simulink model "3-Phase Diode Rectifier"  (R2025a)
settings: Solver=VariableStepAuto  StartTime=0.0  StopTime=100  RelTol=1e-3
values from neighbouring files (symbols this model uses):
  OnTime = (SpikeTime / TimePeriod) * 100    [run_week_6_day_4.m]
  SpikeTime = evalin('base', 'SpikeTime')    [run_week_6_day_4.m]
  TimePeriod = evalin('base', 'TimePeriod')    [run_week_6_day_4.m]
undefined symbols (not defined in the file or in its folder): myFlag
libraries: fl_lib x32, nesl_utility x22, ee_lib x11
settings Model: Creator=adars  LastModifiedBy=adars
settings DebuggingCC: AlgebraicLoopMsg=none

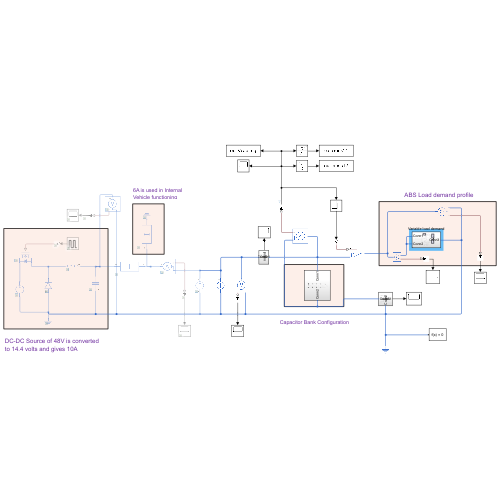
[thumbnail: Simulink's stored preview of the top-level diagram]
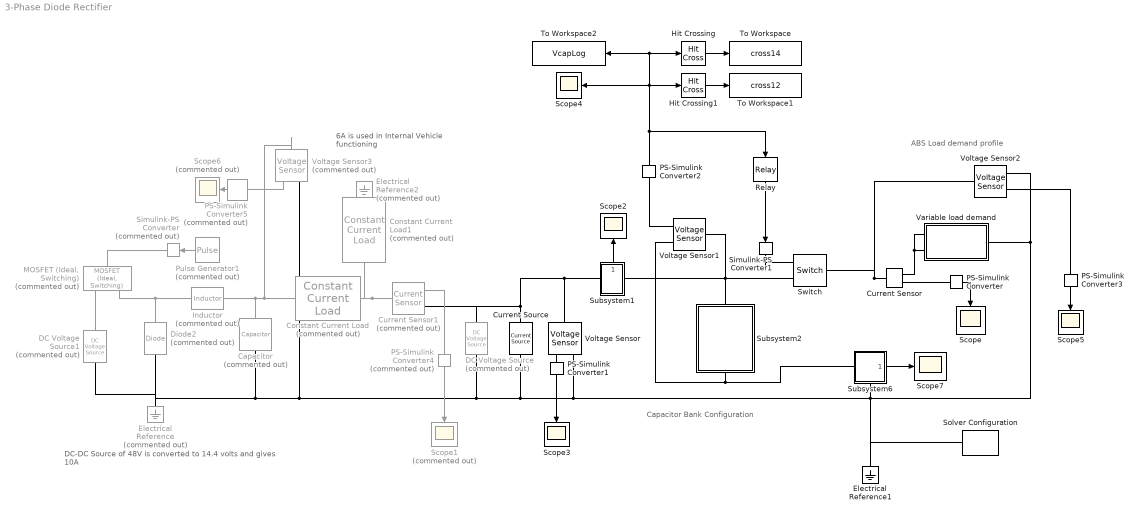
== system 3-Phase Diode Rectifier ==
  note: Capacitor Bank Configuration
  note: ABS Load demand profile
  note: 6A is used in Internal
      | Vehicle functioning
  note: DC-DC Source of 48V is converted
      | to 14.4 volts and gives 10A
  Capacitor : fl_lib/Electrical/Electrical Elements/Capacitor  Commented=on  c=48.3e-6 F  r=1e-6 Ohm  g=0 1/Ohm  i_specify=off  i_priority=None  i=0 A  i_nominal_specify=off  i_nominal_value=1  i_nominal_unit=A  v_specify=off  v_priority=None  v=0 V  v_nominal_specify=off  v_nominal_value=1  v_nominal_unit=V  vc_specify=off  vc_priority=High  vc=0 V  vc_nominal_specify=off  vc_nominal_value=1  vc_nominal_unit=V
  Constant Current Load : ee_lib/Passive/Constant Current Load  Commented=on  load_type=ee.enum.dc_ac.dc  consumed_current=10 A  min_supply_voltage=0.1 V  G_reverse=1e-6 S  deltaV=1e-3 V  consumed_current_rms=100 A  f0=60 Hz  Vrms_min=200 V
      settings: InternalSimscapePortConfiguration="{\"Bottom\":[],\"Left\":[{\"id\":\"p\",\"label\":\"+\",\"type\":\"foundation.electrical.electrical\"}],\"Right\":[{\"id\":\"n\",\"label\":\"-\",\"type\":\"foundation.electrical.electrical\"}],\"Top\":[]}"
  Constant Current Load1 : ee_lib/Passive/Constant Current Load  Commented=on  load_type=ee.enum.dc_ac.dc  consumed_current=6 A  min_supply_voltage=5 V  G_reverse=1e-6 S  deltaV=1e-3 V  consumed_current_rms=100 A  f0=60 Hz  Vrms_min=200 V
      settings: InternalSimscapePortConfiguration="{\"Bottom\":[],\"Left\":[{\"id\":\"p\",\"label\":\"+\",\"type\":\"foundation.electrical.electrical\"}],\"Right\":[{\"id\":\"n\",\"label\":\"-\",\"type\":\"foundation.electrical.electrical\"}],\"Top\":[]}"
  Current Sensor : fl_lib/Electrical/Electrical Sensors/Current Sensor
  Current Sensor1 : fl_lib/Electrical/Electrical Sensors/Current Sensor  Commented=on
  Current Source : ee_lib/Sources/Current Source  dc_current=CurrentSource A  ac_current=0 A  ac_shift=0 rad  ac_frequency=0 Hz  noise_mode=ee.enum.sources.noise.Disabled  PSD=0 A^2/Hz  sample_time=1e-3 s  repeatability=ee.enum.sources.repeatability.NotRepeatable  user_seed=0  auto_seed=3499211588  i_specify=off  i_priority=None  i=0 A  i_nominal_specify=off  i_nominal_value=1  i_nominal_unit=A  v_specify=off  v_priority=None  v=0 V  v_nominal_specify=off  v_nominal_value=1  v_nominal_unit=V
  DC Voltage Source : ee_lib/Additional Components/SPICE Sources/DC Voltage Source  Commented=on  DC=14.4 V
  DC Voltage Source1 : ee_lib/Additional Components/SPICE Sources/DC Voltage Source  Commented=on  DC=48 V
  Diode2 : fl_lib/Electrical/Electrical Elements/Diode  Commented=on  Vf=0.6 V  Ron=0.3 Ohm  Goff=1e-8 1/Ohm  i_specify=off  i_priority=None  i=0 A  i_nominal_specify=off  i_nominal_value=1  i_nominal_unit=A  v_specify=off  v_priority=None  v=0 V  v_nominal_specify=off  v_nominal_value=1  v_nominal_unit=V
  Electrical Reference : fl_lib/Electrical/Electrical Elements/Electrical Reference  Commented=on
  Electrical Reference1 : fl_lib/Electrical/Electrical Elements/Electrical Reference
  Electrical Reference2 : fl_lib/Electrical/Electrical Elements/Electrical Reference  Commented=on
  Hit Crossing : HitCross  HitCrossingOffset=14.4-1e-5  HitCrossingDirection=rising
  Hit Crossing1 : HitCross  HitCrossingOffset=12+1e-5  HitCrossingDirection=falling
  Inductor : ee_lib/Passive/Inductor  Commented=on  l=22e-6 H  enable_L_tol=ee.enum.toleranceApplication.none  L_tol=20  tol_distribution=ee.enum.toleranceDistribution.uniform  nSigma=4  r=0 Ohm  g=1e-9 1/Ohm  enable_operating_limits=ee.enum.enable.no  operating_limit_action=ee.enum.passive.reportOpLim.warn  max_working_current=1 A  power_rating=1 W  i_L_specify=off  i_L_priority=High  i_L=0 A  i_L_nominal_specify=off  i_L_nominal_value=1  i_L_nominal_unit=A
  "MOSFET (Ideal, Switching)" : ee_lib/Semiconductors & Converters/MOSFET (Ideal, Switching)  Commented=on  port_option=ee.enum.controlport.ps  Rds=0.01 Ohm  Goff=1e-6 1/Ohm  Vth=2 V  diode_param=ee.enum.semiconductors.protectionDiode.nodynamics  diode_Vf=0.8 V  diode_Ron=0.001 Ohm  diode_Goff=1e-5 1/Ohm  diode_C=50e-9 F  diode_iRM=-235 A  diode_iF=300 A  diode_idot=-50 A/us  diode_trr_param=ee.enum.converters.diodeReverseParam.trr_factor  diode_trr_factor=3  diode_trr=15 us  diode_Qrr=1500 s*uA  ids_specify=off  ids_priority=None  ids=0 A  ids_nominal_specify=off  ids_nominal_value=1  ids_nominal_unit=A  vds_specify=off  vds_priority=None  vds=0 V  vds_nominal_specify=off  vds_nominal_value=1  vds_nominal_unit=V  vgs_specify=off  vgs_priority=None  vgs=0 V  vgs_nominal_specify=off  vgs_nominal_value=1  vgs_nominal_unit=V  thermal_loss_option=ee.enum.converters.thermalLossOption.constantvalues  Von_data=[0, 1.8, 3.2, 6, 10, 16; 0, 2, 5.5, 9.5, 15, 25] V  Tj=[298.15, 448.15] K  Iout_data=[0, 20, 40, 60, 80, 100] A  Eon_data=[0, 55.04, 124.57, 235.53, 362.12; 0, 71.25, 161.25, 304.88, 468.75] * 1e-6 J  Eoff_data=[0, 18, 30, 56.1, 76.5; 0, 22.5, 37.5, 70.13, 95.63] * 1e-6 J  Eon_data_3D=[zeros(2, 5, 3)] J  Eoff_data_3D=[zeros(2, 5, 3)] J  Tj_loss=[298.15, 448.15] K  Iout_data_loss=[0, 10, 20, 30, 40] A  tabulateWithVds=false  Vds_loss=[0, 150, 300] V  Eon_scalar=22.86e-3 J  Eoff_scalar=17.14e-3 J  Voff=300 V  Iout_scalar=600 A  useCurrentFromPreviousCycle=false  useVoltageFromPreviousCycle=false  diodeModelType=ee.enum.converters.diodeModelType.pwl  diodeTableType=ee.enum.diode.tableType.IfMat  diode_ReverseIVType=ee.enum.diode.diodeReverseIV.constant  diode_IfMat=[.07, .12, .19, 1.75, 4.24, 7.32, 11.2; .16, .3, .72, 2.14, 4.02, 6.35, 9.12] A  diode_VfMat=[.9, 1.15, 1.25, 1.5, 1.75, 2.17, 2.6, 2.85; .58, .68, .75, 1.1, 1.38, 1.77, 2.27, 2.7] V  diode_TjVec=[25, 125] degC  diode_VfVec=[.5, .7, .9, 1.3, 1.7, 2.1, 2.5] V  diode_IfVec=[.1, .2, .5, 1, 2, 4, 7, 10] A  diode_IrMat=[1e-06, 2e-06, 5e-06, 1e-05, 2.5e-05, 5e-05, .0001; 2e-06, 5e-06, 1e-05, 4e-05, 8e-05, .0002, .0005] A  diode_VrMat=[10, 100, 200, 250, 300, 325, 350; 10, 70, 160, 220, 270, 300, 320] V  diode_VrVec=[10, 20, 40, 50, 70, 80, 100] V  diode_IrVec=[1e-06, 2e-06, 5e-06, 1e-05, 2e-05, 5e-05, .0001] A  diode_Vr=-600 V  diode_Ls=150 nH  diode_Erec=0.03 J  diode_rec_loss_model=ee.enum.diode.reverseRecoveryModel.fixed  diode_ErecVal=0 J  diode_scaleWithIandV=true  diode_ErecMat=zeros(2, 3) J  diode_TjrecVec=[298.15, 398.15] K  diode_IfrecVec=[.1, 1, 10] A  diode_IrecVal=10 A  diode_VrecVal=10 V  diode_tFilter=1 / 1000 / 100 s  separateThermalPortForDiode=false  thermal_network_parameterization=ee.enum.thermalNetworkTopology.external  Rth=[.03, .2] K/W  Rth_Cauer=[.03, .1, .2] K/W  Rth_Foster=[.08, .14, .22, .16] K/W  thermal_mass_parameterization=ee.enum.thermalNetwork.timeconstant  thermal_mass=[3, 25] J/K  thermal_mass_Cauer=[3, 10, 25] J/K  thermal_mass_Foster=[.001, .005, .05, .5] J/K  thermal_time_constant=[.1, 5] s  thermal_time_constant_Cauer=[.1, 1, 5] s  thermal_time_constant_Foster=[7e-05, .0007, .01, .08] s  thermal_mass_initial_temperatures=[25, 25] degC  thermal_mass_initial_temperatures_Cauer=[25, 25, 25] degC  junction_thermal_mass=0.1 J/K  Tvec_initial_Foster=[25, 25, 25, 25] degC  RthDiode=[.03, .2] K/W  RthCauerDiode=[.03, .1, .2] K/W  RthFosterDiode=[.03, .2] K/W  thermalMassDiode=[3, 25] J/K  thermalMassCauerDiode=[3, 10, 25] J/K  thermalMassFosterDiode=[33, 50] J/K  thermalTauDiode=[.1, 5] s  thermalTauCauerDiode=[.1, 1, 5] s  thermalTauFosterDiode=[1, 10] s  thermalMassInitTempDiode=[25, 25] degC  thermalMassInitTempCauerDiode=[25, 25, 25] degC  junctionthermalMassDiode=0.1 J/K  TVecInitialFosterDiode=[25, 25, 25, 25] degC  no_thermal_network=0  mosfet_junction_temperature_specify=off  mosfet_junction_temperature_priority=None  mosfet_junction_temperature=25 degC  mosfet_junction_temperature_nominal_specify=off  mosfet_junction_temperature_nominal_value=1  mosfet_junction_temperature_nominal_unit=degC  diode_junction_temperature_specify=off  diode_junction_temperature_priority=None  diode_junction_temperature=25 degC  diode_junction_temperature_nominal_specify=off  diode_junction_temperature_nominal_value=1  diode_junction_temperature_nominal_unit=degC  Qj_specify=off  Qj_priority=None  Qj=0 W  Qj_nominal_specify=off  Qj_nominal_value=1  Qj_nominal_unit=W  accumulatedSwitchingLosses_specify=off  accumulatedSwitchingLosses_priority=None  accumulatedSwitchingLosses=0 J
  PS-Simulink Converter{,1..3} (4 alike) : nesl_utility/PS-Simulink Converter  PhysicalDomain=network_engine_domain  SubClassName=ps_output  LeftPortType=input  RightPortType=output  PseudoPeriodic=off  Frequencies=[]  VectorFormat=inherit  Unit=inherit  AffineConversion=off
  PS-Simulink Converter4 : nesl_utility/PS-Simulink Converter  Commented=on  PhysicalDomain=network_engine_domain  SubClassName=ps_output  LeftPortType=input  RightPortType=output  PseudoPeriodic=off  Frequencies=[]  VectorFormat=inherit  Unit=inherit  AffineConversion=off
  PS-Simulink Converter5 : nesl_utility/PS-Simulink Converter  Commented=on  PhysicalDomain=network_engine_domain  SubClassName=ps_output  LeftPortType=input  RightPortType=output  PseudoPeriodic=off  Frequencies=[]  VectorFormat=inherit  Unit=inherit  AffineConversion=off
  Pulse Generator1 : DiscretePulseGenerator  Commented=on  PulseType=Time based  Amplitude=10  Period=6.8e-6  PulseWidth=35
  Relay : Relay  OnSwitchValue=14.4  OffSwitchValue=12
  Scope{,2..5,7} (6 alike) : Scope
      Scope settings: ActiveDisplayYMinimum=-1.307559668572738  ActiveDisplayYMaximum=0.60259783482282581
      Scope2 settings: ActiveDisplayYMinimum=3  ActiveDisplayYMaximum=5  DataLoggingVariableName=ScopeData2
      Scope3 settings: ActiveDisplayYMinimum=-1.84775774004581  ActiveDisplayYMaximum=16.629859660412297  DataLoggingVariableName=ScopeData3
      Scope4 settings: ActiveDisplayYMinimum=11.713414975625813  ActiveDisplayYMaximum=13.359784553943715  DataLoggingVariableName=ScopeData4
      Scope5 settings: ActiveDisplayYMinimum=-1.2935840970910446  ActiveDisplayYMaximum=16.143708233009956  DataLoggingVariableName=ScopeData5
      Scope7 settings: ActiveDisplayYMinimum=-24.12500014418708  ActiveDisplayYMaximum=7.1249998826875194  DataLoggingVariableName=ScopeData13
  Scope1 : Scope  Commented=on
      settings: ActiveDisplayYMinimum=-7.2502393778438039  ActiveDisplayYMaximum=5.2520104006562276  DataLoggingVariableName=ScopeData10
  Scope6 : Scope  Commented=on
      settings: ActiveDisplayYMinimum=-2.4456957415230445  ActiveDisplayYMaximum=22.011261673851934  DataLoggingVariableName=ScopeData14
  Simulink-PS Converter : nesl_utility/Simulink-PS Converter  Commented=on  PhysicalDomain=network_engine_domain  SubClassName=ps_input  LeftPortType=input  RightPortType=output  PseudoPeriodic=off  Frequencies=[]  NoiseDistribution=none  NoiseParameters=[]  Unit=1  AffineConversion=off  FilteringAndDerivatives=provide  SimscapeFilterOrder=1  InputFilterTimeConstant=0.001  UdotUserProvided=0
  Simulink-PS Converter1 : nesl_utility/Simulink-PS Converter  PhysicalDomain=network_engine_domain  SubClassName=ps_input  LeftPortType=input  RightPortType=output  PseudoPeriodic=off  Frequencies=[]  NoiseDistribution=none  NoiseParameters=[]  Unit=1  AffineConversion=off  FilteringAndDerivatives=provide  SimscapeFilterOrder=1  InputFilterTimeConstant=0.001  UdotUserProvided=0
  Solver Configuration : nesl_utility/Solver Configuration  PhysicalDomain=network_engine_domain  SubClassName=solver  LeftPortType=input  RightPortType=generic  Tones=[]  Harmonics=[]  SimulateNoise=off  Profile=off  UseLocalSampling=off  EnableSwitchedLinearOptims=on  FrequencyDomain=off  UseCCode=off  RelTol=0.001  AbsTol=0.001  MinStep=1e-09  ToWorkspace=off  RevertToSquareIcSolve=off  NumHomotopyIterations=100  PhasorMode=off  PhasorModeNumHarmonics=1  ConsistencySolver=NEWTON_XTOL_AFTER_FTOL  IndexReductionMethod=DerivativeReplacement  DoDC=off  ResidualTolerance=1e-09  ConsistencyTolSource=GLOBAL  ConsistencyAbsTol=0.001  ConsistencyRelTol=0.001  ConsistencyTolFactor=0.001  UseLocalSolver=off  LocalSolverChoice=NE_BACKWARD_EULER_ADVANCER  ResolveIndetEquations=on  FunctionEvalNumThread=1  LocalSolverSampleTime=0.001  DoFixedCost=off  MaxNonlinIter=3  MaxModeIter=2  ComputeImpulses=off  ImpulseIterations=2  LinearAlgebra=auto  LinearAlgebraNumThread=0  EquationFormulation=NE_TIME_EF  DelaysMemoryBudget=1024  AutomaticFiltering=on  FilteringTimeConstant=0.001  PartitionStorageMethod=AS_NEEDED  PartitionMemoryBudget=1024  PartitionMethod=ROBUST  MultibodyUseLocalSolver=off  MultibodyLocalSolverChoice=ODE1  MultibodyLocalSolverSampleTime=0.001
  Subsystem1 : Subsystem
      settings: PortSchema="{\"entries\":[{\"content\":{\"sides\":[{\"content\":{\"connectorIds\":[\"LConn1\"]},\"type\":\"ConnectorPlacement.EquallySpacedRectSide\",\"uuid\":\"0bfba3d8-eada-431e-8566-6f8409c961ce\"},{\"content\":{\"connectorIds\":[\"RConn1\"],\"side\":\"RIGHT\"},\"type\":\"ConnectorPlacement.EquallySpacedRectSide\",\"uuid\":\"a4875283-c2aa-4032-81af-fd742f95824b\"},{\"content\":{\"connectorIds\":[\"Out1\"],\"side\":\"TOP\"},\"type\":\"ConnectorPlacement.EquallySpacedRectSide\",\"uuid\":\"06f00768-eb41-4938-823b-845aa4a9ac6f\"}]},\"type\":\"ConnectorPlacement.EquallySpacedConnector\",\"uuid\":\"d87aa723-8170-4005-95e2-aec9f879c413\"}],\"packageUris\":[\"http://schema.mathworks.com/mf0/Connector/R2020b\"],\"version\":\"1.0\"}"
  Subsystem2 : Subsystem
  Subsystem6 : Subsystem
      settings: PortSchema="{\"entries\":[{\"content\":{\"sides\":[{\"content\":{\"connectorIds\":[\"LConn1\"]},\"type\":\"ConnectorPlacement.EquallySpacedRectSide\",\"uuid\":\"0bfba3d8-eada-431e-8566-6f8409c961ce\"},{\"content\":{\"connectorIds\":[\"Out1\"],\"side\":\"RIGHT\"},\"type\":\"ConnectorPlacement.EquallySpacedRectSide\",\"uuid\":\"a4875283-c2aa-4032-81af-fd742f95824b\"},{\"content\":{\"side\":\"TOP\"},\"type\":\"ConnectorPlacement.EquallySpacedRectSide\",\"uuid\":\"06f00768-eb41-4938-823b-845aa4a9ac6f\"},{\"content\":{\"connectorIds\":[\"RConn1\"],\"side\":\"BOTTOM\"},\"type\":\"ConnectorPlacement.EquallySpacedRectSide\",\"uuid\":\"36f95f34-d0b9-4c5e-948a-2f9aa4eedbf8\"}]},\"type\":\"ConnectorPlacement.EquallySpacedConnector\",\"uuid\":\"d87aa723-8170-4005-95e2-aec9f879c413\"}],\"packageUris\":[\"http://schema.mathworks.com/mf0/Connector/R2020b\"],\"version\":\"1.0\"}"
  Switch : fl_lib/Electrical/Electrical Elements/Switch  R_closed=0.01 Ohm  G_open=1e-8 1/Ohm  Threshold=0.5  i_specify=off  i_priority=None  i=0 A  i_nominal_specify=off  i_nominal_value=1  i_nominal_unit=A  v_specify=off  v_priority=None  v=0 V  v_nominal_specify=off  v_nominal_value=1  v_nominal_unit=V
  To Workspace : ToWorkspace  VariableName=cross14  SampleTime=-1
  To Workspace1 : ToWorkspace  VariableName=cross12  SampleTime=-1
  To Workspace2 : ToWorkspace  VariableName=VcapLog  SaveFormat=Timeseries  SampleTime=-1
  Variable load demand : Subsystem
  Voltage Sensor : fl_lib/Electrical/Electrical Sensors/Voltage Sensor
  Voltage Sensor1 : fl_lib/Electrical/Electrical Sensors/Voltage Sensor
  Voltage Sensor2 : fl_lib/Electrical/Electrical Sensors/Voltage Sensor
  Voltage Sensor3 : fl_lib/Electrical/Electrical Sensors/Voltage Sensor  Commented=on
  wires:
  PS-Simulink Converter3/1 -> Scope5/1
  PS-Simulink Converter/1 -> Scope/1
  PS-Simulink Converter5/1 -> Scope6/1
  PS-Simulink Converter1/1 -> Scope3/1
  Pulse Generator1/1 -> Simulink-PS Converter/1
  PS-Simulink Converter2/1 -> Scope4/1, To Workspace2/1, Hit Crossing/1, Hit Crossing1/1, Relay/1
  Hit Crossing1/1 -> To Workspace1/1
  Subsystem1/1(output) -> Scope2/1
  Subsystem6/1(output) -> Scope7/1
  PS-Simulink Converter4/1 -> Scope1/1
  Relay/1 -> Simulink-PS Converter1/1
  Hit Crossing/1 -> To Workspace/1
  connections:
  Voltage Sensor1/LConn1 -- Subsystem1/RConn1 -- Subsystem2/LConn1 -- Switch/RConn2
  Current Sensor/LConn1 -- Switch/LConn1 -- Voltage Sensor2/LConn1
  Diode2/RConn1 -- "MOSFET (Ideal, Switching)"/RConn2 -- Inductor/LConn1
  Constant Current Load1/LConn1 -- Constant Current Load/RConn1 -- Current Sensor1/LConn1
  Voltage Sensor3/LConn1 -- Capacitor/LConn1 -- Inductor/RConn1 -- Constant Current Load/LConn1
  Current Source/RConn1 -- Voltage Sensor3/RConn2 -- DC Voltage Source1/RConn1 -- Electrical Reference/LConn1 -- Diode2/LConn1 -- Capacitor/RConn1 -- DC Voltage Source/RConn1 -- Solver Configuration/RConn1 -- Electrical Reference1/LConn1 -- Subsystem6/RConn1 -- Voltage Sensor2/RConn2 -- Variable load demand/LConn1 -- Voltage Sensor/RConn2
  Voltage Sensor/LConn1 -- Current Sensor1/RConn2 -- DC Voltage Source/LConn1 -- Current Source/LConn1 -- Subsystem1/LConn1
  Voltage Sensor1/RConn2 -- Subsystem2/RConn1 -- Subsystem6/LConn1
  Current Sensor/RConn2 -- Variable load demand/RConn2 -- Variable load demand/RConn1
  PS-Simulink Converter1/LConn1 -- Voltage Sensor/RConn1
  PS-Simulink Converter2/LConn1 -- Voltage Sensor1/RConn1
  DC Voltage Source1/LConn1 -- "MOSFET (Ideal, Switching)"/RConn1
  PS-Simulink Converter/LConn1 -- Current Sensor/RConn1
  PS-Simulink Converter5/LConn1 -- Voltage Sensor3/RConn1
  Simulink-PS Converter/RConn1 -- "MOSFET (Ideal, Switching)"/LConn1
  Simulink-PS Converter1/RConn1 -- Switch/RConn1
  Constant Current Load1/RConn1 -- Electrical Reference2/LConn1
  Current Sensor1/RConn1 -- PS-Simulink Converter4/LConn1
  PS-Simulink Converter3/LConn1 -- Voltage Sensor2/RConn1

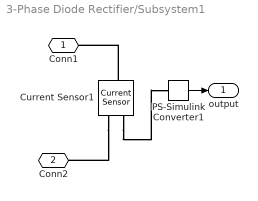
== system 3-Phase Diode Rectifier/Subsystem1 ==
  Current Sensor1 : fl_lib/Electrical/Electrical Sensors/Current Sensor
  PS-Simulink Converter1 : nesl_utility/PS-Simulink Converter  PhysicalDomain=network_engine_domain  SubClassName=ps_output  LeftPortType=input  RightPortType=output  PseudoPeriodic=off  Frequencies=[]  VectorFormat=inherit  Unit=inherit  AffineConversion=off
  Conn1 : PMIOPort  Side=Left
  Conn2 : PMIOPort  Port=2  Side=Right
  output : Outport
  wires:
  PS-Simulink Converter1/1 -> output/1
  connections:
  Current Sensor1/RConn1 -- PS-Simulink Converter1/LConn1
  Current Sensor1/LConn1 -- Conn1/RConn1
  Current Sensor1/RConn2 -- Conn2/RConn1

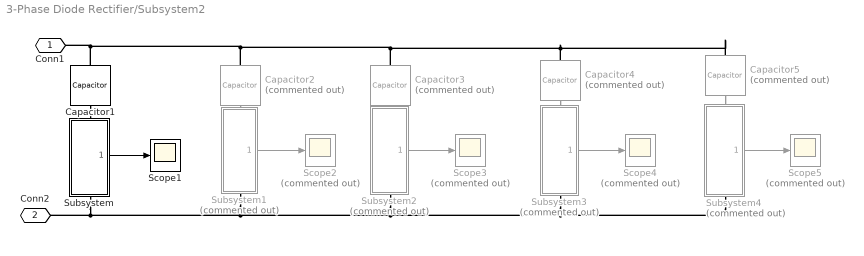
== system 3-Phase Diode Rectifier/Subsystem2 ==
  Capacitor1 : fl_lib/Electrical/Electrical Elements/Capacitor  c=C_val F  r=1e-6 Ohm  g=0 1/Ohm  i_specify=off  i_priority=None  i=0 A  i_nominal_specify=off  i_nominal_value=1  i_nominal_unit=A  v_specify=off  v_priority=None  v=0 V  v_nominal_specify=off  v_nominal_value=1  v_nominal_unit=V  vc_specify=on  vc_priority=High  vc=12 V  vc_nominal_specify=off  vc_nominal_value=1  vc_nominal_unit=V
  Capacitor{2..5} (4 alike) : fl_lib/Electrical/Electrical Elements/Capacitor  Commented=on  c=22.5 F  r=1e-6 Ohm  g=0 1/Ohm  i_specify=off  i_priority=None  i=0 A  i_nominal_specify=off  i_nominal_value=1  i_nominal_unit=A  v_specify=off  v_priority=None  v=0 V  v_nominal_specify=off  v_nominal_value=1  v_nominal_unit=V  vc_specify=on  vc_priority=High  vc=12 V  vc_nominal_specify=off  vc_nominal_value=1  vc_nominal_unit=V
  Scope1 : Scope
      settings: ActiveDisplayYMinimum=-32.03150883871016  ActiveDisplayYMaximum=5.6799472599220806
  Scope{2..5} (4 alike) : Scope  Commented=on
      Scope2 settings: ActiveDisplayYMinimum=-32.03150883871016  ActiveDisplayYMaximum=5.6799472599220806  DataLoggingVariableName=ScopeData6
      Scope3 settings: ActiveDisplayYMinimum=-32.03150883871016  ActiveDisplayYMaximum=5.6799472599220806  DataLoggingVariableName=ScopeData7
      Scope4 settings: ActiveDisplayYMinimum=-32.03150883871016  ActiveDisplayYMaximum=5.6799472599220806  DataLoggingVariableName=ScopeData8
      Scope5 settings: ActiveDisplayYMinimum=-32.03150883871016  ActiveDisplayYMaximum=5.6799472599220806  DataLoggingVariableName=ScopeData9
  Subsystem : Subsystem
      settings: PortSchema="{\"entries\":[{\"content\":{\"sides\":[{\"content\":{\"connectorIds\":[\"LConn1\"]},\"type\":\"ConnectorPlacement.EquallySpacedRectSide\",\"uuid\":\"81a8c0f4-8ed9-4d4b-bd28-04771a05fe4f\"},{\"content\":{\"connectorIds\":[\"RConn1\"],\"side\":\"RIGHT\"},\"type\":\"ConnectorPlacement.EquallySpacedRectSide\",\"uuid\":\"31ca84c7-3f86-4e13-8cf7-6dd391f2d0e6\"},{\"content\":{\"connectorIds\":[\"Out1\"],\"side\":\"TOP\"},\"type\":\"ConnectorPlacement.EquallySpacedRectSide\",\"uuid\":\"282c2d81-43af-474c-80bd-93514e90c90d\"}]},\"type\":\"ConnectorPlacement.EquallySpacedConnector\",\"uuid\":\"f82acd1c-4042-44ca-a2b0-ecaad96ae19c\"}],\"packageUris\":[\"http://schema.mathworks.com/mf0/Connector/R2020b\"],\"version\":\"1.0\"}"
  Subsystem1 : Subsystem  Commented=on
      settings: PortSchema="{\"entries\":[{\"content\":{\"sides\":[{\"content\":{\"connectorIds\":[\"LConn1\"]},\"type\":\"ConnectorPlacement.EquallySpacedRectSide\",\"uuid\":\"81a8c0f4-8ed9-4d4b-bd28-04771a05fe4f\"},{\"content\":{\"connectorIds\":[\"RConn1\"],\"side\":\"RIGHT\"},\"type\":\"ConnectorPlacement.EquallySpacedRectSide\",\"uuid\":\"31ca84c7-3f86-4e13-8cf7-6dd391f2d0e6\"},{\"content\":{\"connectorIds\":[\"Out1\"],\"side\":\"TOP\"},\"type\":\"ConnectorPlacement.EquallySpacedRectSide\",\"uuid\":\"282c2d81-43af-474c-80bd-93514e90c90d\"}]},\"type\":\"ConnectorPlacement.EquallySpacedConnector\",\"uuid\":\"f82acd1c-4042-44ca-a2b0-ecaad96ae19c\"}],\"packageUris\":[\"http://schema.mathworks.com/mf0/Connector/R2020b\"],\"version\":\"1.0\"}"
  Subsystem2 : Subsystem  Commented=on
      settings: PortSchema="{\"entries\":[{\"content\":{\"sides\":[{\"content\":{\"connectorIds\":[\"LConn1\"]},\"type\":\"ConnectorPlacement.EquallySpacedRectSide\",\"uuid\":\"81a8c0f4-8ed9-4d4b-bd28-04771a05fe4f\"},{\"content\":{\"connectorIds\":[\"RConn1\"],\"side\":\"RIGHT\"},\"type\":\"ConnectorPlacement.EquallySpacedRectSide\",\"uuid\":\"31ca84c7-3f86-4e13-8cf7-6dd391f2d0e6\"},{\"content\":{\"connectorIds\":[\"Out1\"],\"side\":\"TOP\"},\"type\":\"ConnectorPlacement.EquallySpacedRectSide\",\"uuid\":\"282c2d81-43af-474c-80bd-93514e90c90d\"}]},\"type\":\"ConnectorPlacement.EquallySpacedConnector\",\"uuid\":\"f82acd1c-4042-44ca-a2b0-ecaad96ae19c\"}],\"packageUris\":[\"http://schema.mathworks.com/mf0/Connector/R2020b\"],\"version\":\"1.0\"}"
  Subsystem3 : Subsystem  Commented=on
      settings: PortSchema="{\"entries\":[{\"content\":{\"sides\":[{\"content\":{\"connectorIds\":[\"LConn1\"]},\"type\":\"ConnectorPlacement.EquallySpacedRectSide\",\"uuid\":\"81a8c0f4-8ed9-4d4b-bd28-04771a05fe4f\"},{\"content\":{\"connectorIds\":[\"RConn1\"],\"side\":\"RIGHT\"},\"type\":\"ConnectorPlacement.EquallySpacedRectSide\",\"uuid\":\"31ca84c7-3f86-4e13-8cf7-6dd391f2d0e6\"},{\"content\":{\"connectorIds\":[\"Out1\"],\"side\":\"TOP\"},\"type\":\"ConnectorPlacement.EquallySpacedRectSide\",\"uuid\":\"282c2d81-43af-474c-80bd-93514e90c90d\"}]},\"type\":\"ConnectorPlacement.EquallySpacedConnector\",\"uuid\":\"f82acd1c-4042-44ca-a2b0-ecaad96ae19c\"}],\"packageUris\":[\"http://schema.mathworks.com/mf0/Connector/R2020b\"],\"version\":\"1.0\"}"
  Subsystem4 : Subsystem  Commented=on
      settings: PortSchema="{\"entries\":[{\"content\":{\"sides\":[{\"content\":{\"connectorIds\":[\"LConn1\"]},\"type\":\"ConnectorPlacement.EquallySpacedRectSide\",\"uuid\":\"81a8c0f4-8ed9-4d4b-bd28-04771a05fe4f\"},{\"content\":{\"connectorIds\":[\"RConn1\"],\"side\":\"RIGHT\"},\"type\":\"ConnectorPlacement.EquallySpacedRectSide\",\"uuid\":\"31ca84c7-3f86-4e13-8cf7-6dd391f2d0e6\"},{\"content\":{\"connectorIds\":[\"Out1\"],\"side\":\"TOP\"},\"type\":\"ConnectorPlacement.EquallySpacedRectSide\",\"uuid\":\"282c2d81-43af-474c-80bd-93514e90c90d\"}]},\"type\":\"ConnectorPlacement.EquallySpacedConnector\",\"uuid\":\"f82acd1c-4042-44ca-a2b0-ecaad96ae19c\"}],\"packageUris\":[\"http://schema.mathworks.com/mf0/Connector/R2020b\"],\"version\":\"1.0\"}"
  Conn1 : PMIOPort  Side=Left
  Conn2 : PMIOPort  Port=2  Side=Right
  wires:
  Subsystem/1(output) -> Scope1/1
  Subsystem1/1(output) -> Scope2/1
  Subsystem2/1(output) -> Scope3/1
  Subsystem3/1(output) -> Scope4/1
  Subsystem4/1(output) -> Scope5/1
  connections:
  Capacitor1/RConn1 -- Subsystem/LConn1
  Capacitor1/LConn1 -- Capacitor5/LConn1 -- Capacitor4/LConn1 -- Capacitor3/LConn1 -- Capacitor2/LConn1 -- Conn1/RConn1
  Subsystem/RConn1 -- Subsystem2/RConn1 -- Subsystem3/RConn1 -- Subsystem4/RConn1 -- Subsystem1/RConn1 -- Conn2/RConn1
  Capacitor2/RConn1 -- Subsystem1/LConn1
  Capacitor3/RConn1 -- Subsystem2/LConn1
  Capacitor4/RConn1 -- Subsystem3/LConn1
  Capacitor5/RConn1 -- Subsystem4/LConn1

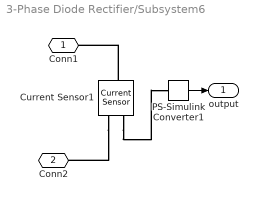
== system 3-Phase Diode Rectifier/Subsystem6 ==
  Current Sensor1 : fl_lib/Electrical/Electrical Sensors/Current Sensor
  PS-Simulink Converter1 : nesl_utility/PS-Simulink Converter  PhysicalDomain=network_engine_domain  SubClassName=ps_output  LeftPortType=input  RightPortType=output  PseudoPeriodic=off  Frequencies=[]  VectorFormat=inherit  Unit=inherit  AffineConversion=off
  Conn1 : PMIOPort  Side=Left
  Conn2 : PMIOPort  Port=2  Side=Right
  output : Outport
  wires:
  PS-Simulink Converter1/1 -> output/1
  connections:
  Current Sensor1/RConn1 -- PS-Simulink Converter1/LConn1
  Current Sensor1/LConn1 -- Conn1/RConn1
  Current Sensor1/RConn2 -- Conn2/RConn1

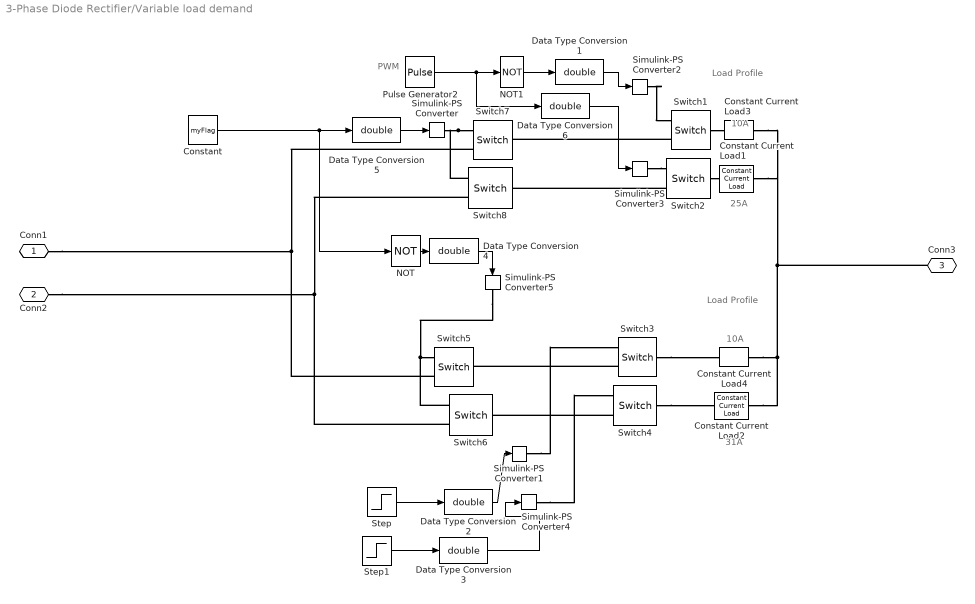
== system 3-Phase Diode Rectifier/Variable load demand ==
  note: 10A
  note: PWM
  note: 25A
  note: 10A
  note: Load Profile
  note: Load Profile
  note: 31A
  Constant : Constant  Value=myFlag
  Constant Current Load1 : ee_lib/Passive/Constant Current Load  load_type=ee.enum.dc_ac.dc  consumed_current=high_current A  min_supply_voltage=1 V  G_reverse=1e-6 S  deltaV=1e-3 V  consumed_current_rms=100 A  f0=60 Hz  Vrms_min=200 V
      settings: InternalSimscapePortConfiguration="{\"Bottom\":[],\"Left\":[{\"id\":\"p\",\"label\":\"+\",\"type\":\"foundation.electrical.electrical\"}],\"Right\":[{\"id\":\"n\",\"label\":\"-\",\"type\":\"foundation.electrical.electrical\"}],\"Top\":[]}"
  Constant Current Load2 : ee_lib/Passive/Constant Current Load  load_type=ee.enum.dc_ac.dc  consumed_current=high_current A  min_supply_voltage=1 V  G_reverse=1e-6 S  deltaV=1e-3 V  consumed_current_rms=100 A  f0=60 Hz  Vrms_min=200 V
      settings: InternalSimscapePortConfiguration="{\"Bottom\":[],\"Left\":[{\"id\":\"p\",\"label\":\"+\",\"type\":\"foundation.electrical.electrical\"}],\"Right\":[{\"id\":\"n\",\"label\":\"-\",\"type\":\"foundation.electrical.electrical\"}],\"Top\":[]}"
  Constant Current Load3 : ee_lib/Passive/Constant Current Load  load_type=ee.enum.dc_ac.dc  consumed_current=low_current A  min_supply_voltage=1 V  G_reverse=1e-6 S  deltaV=1e-3 V  consumed_current_rms=100 A  f0=60 Hz  Vrms_min=200 V
      settings: InternalSimscapePortConfiguration="{\"Bottom\":[],\"Left\":[{\"id\":\"p\",\"label\":\"+\",\"type\":\"foundation.electrical.electrical\"}],\"Right\":[{\"id\":\"n\",\"label\":\"-\",\"type\":\"foundation.electrical.electrical\"}],\"Top\":[]}"
  Constant Current Load4 : ee_lib/Passive/Constant Current Load  load_type=ee.enum.dc_ac.dc  consumed_current=low_current A  min_supply_voltage=1 V  G_reverse=1e-6 S  deltaV=1e-3 V  consumed_current_rms=100 A  f0=60 Hz  Vrms_min=200 V
      settings: InternalSimscapePortConfiguration="{\"Bottom\":[],\"Left\":[{\"id\":\"p\",\"label\":\"+\",\"type\":\"foundation.electrical.electrical\"}],\"Right\":[{\"id\":\"n\",\"label\":\"-\",\"type\":\"foundation.electrical.electrical\"}],\"Top\":[]}"
  Data Type Conversion{1..6} (6 alike) : DataTypeConversion  OutDataTypeStr=double  SaturateOnIntegerOverflow=off  RndMeth=Floor
  NOT : Logic  Operator=NOT  IconShape=distinctive  AllPortsSameDT=off  OutDataTypeStr=boolean
  NOT1 : Logic  Operator=NOT  IconShape=distinctive  AllPortsSameDT=off  OutDataTypeStr=boolean
  Pulse Generator2 : DiscretePulseGenerator  PulseType=Time based  Period=TimePeriod  PulseWidth=OnTime
  Simulink-PS Converter{,1..5} (6 alike) : nesl_utility/Simulink-PS Converter  PhysicalDomain=network_engine_domain  SubClassName=ps_input  LeftPortType=input  RightPortType=output  PseudoPeriodic=off  Frequencies=[]  NoiseDistribution=none  NoiseParameters=[]  Unit=1  AffineConversion=off  FilteringAndDerivatives=provide  SimscapeFilterOrder=1  InputFilterTimeConstant=0.001  UdotUserProvided=0
  Step : Step  Time=SpikeTime  SampleTime=0
  Step1 : Step  Time=SpikeTime  Before=1  After=0  SampleTime=0
  Switch{1..8} (8 alike) : fl_lib/Electrical/Electrical Elements/Switch  R_closed=0.01 Ohm  G_open=1e-8 1/Ohm  Threshold=0.5  i_specify=off  i_priority=None  i=0 A  i_nominal_specify=off  i_nominal_value=1  i_nominal_unit=A  v_specify=off  v_priority=None  v=0 V  v_nominal_specify=off  v_nominal_value=1  v_nominal_unit=V
  Conn1 : PMIOPort  Side=Right
  Conn2 : PMIOPort  Port=2  Side=Right
  Conn3 : PMIOPort  Port=3  Side=Left
  wires:
  Data Type Conversion2/1 -> Simulink-PS Converter1/1
  Pulse Generator2/1 -> Data Type Conversion6/1, NOT1/1
  Step1/1 -> Data Type Conversion3/1
  Data Type Conversion4/1 -> Simulink-PS Converter5/1
  NOT/1 -> Data Type Conversion4/1
  Data Type Conversion6/1 -> Simulink-PS Converter3/1
  NOT1/1 -> Data Type Conversion1/1
  Data Type Conversion5/1 -> Simulink-PS Converter/1
  Data Type Conversion1/1 -> Simulink-PS Converter2/1
  Step/1 -> Data Type Conversion2/1
  Data Type Conversion3/1 -> Simulink-PS Converter4/1
  Constant/1 -> Data Type Conversion5/1, NOT/1
  connections:
  Switch6/RConn2 -- Conn2/RConn1 -- Switch8/RConn2
  Switch5/RConn2 -- Conn1/RConn1 -- Switch7/RConn2
  Constant Current Load4/RConn1 -- Constant Current Load2/RConn1 -- Conn3/RConn1 -- Constant Current Load1/RConn1 -- Constant Current Load3/RConn1
  Simulink-PS Converter/RConn1 -- Switch7/RConn1 -- Switch8/RConn1
  Switch6/RConn1 -- Switch5/RConn1 -- Simulink-PS Converter5/RConn1
  Simulink-PS Converter1/RConn1 -- Switch3/RConn1
  Simulink-PS Converter3/RConn1 -- Switch2/RConn1
  Switch2/LConn1 -- Constant Current Load1/LConn1
  Simulink-PS Converter4/RConn1 -- Switch4/RConn1
  Switch1/LConn1 -- Constant Current Load3/LConn1
  Switch4/RConn2 -- Switch6/LConn1
  Switch3/LConn1 -- Constant Current Load4/LConn1
  Simulink-PS Converter2/RConn1 -- Switch1/RConn1
  Switch2/RConn2 -- Switch8/LConn1
  Switch4/LConn1 -- Constant Current Load2/LConn1
  Switch3/RConn2 -- Switch5/LConn1
  Switch1/RConn2 -- Switch7/LConn1

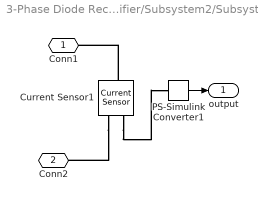
== system 3-Phase Diode Rectifier/Subsystem2/Subsystem ==
  Current Sensor1 : fl_lib/Electrical/Electrical Sensors/Current Sensor
  PS-Simulink Converter1 : nesl_utility/PS-Simulink Converter  PhysicalDomain=network_engine_domain  SubClassName=ps_output  LeftPortType=input  RightPortType=output  PseudoPeriodic=off  Frequencies=[]  VectorFormat=inherit  Unit=inherit  AffineConversion=off
  Conn1 : PMIOPort  Side=Left
  Conn2 : PMIOPort  Port=2  Side=Right
  output : Outport
  wires:
  PS-Simulink Converter1/1 -> output/1
  connections:
  Current Sensor1/RConn1 -- PS-Simulink Converter1/LConn1
  Current Sensor1/LConn1 -- Conn1/RConn1
  Current Sensor1/RConn2 -- Conn2/RConn1

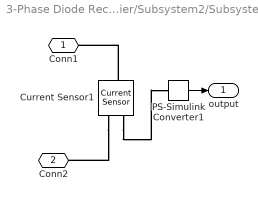
== system 3-Phase Diode Rectifier/Subsystem2/Subsystem1 ==
  Current Sensor1 : fl_lib/Electrical/Electrical Sensors/Current Sensor
  PS-Simulink Converter1 : nesl_utility/PS-Simulink Converter  PhysicalDomain=network_engine_domain  SubClassName=ps_output  LeftPortType=input  RightPortType=output  PseudoPeriodic=off  Frequencies=[]  VectorFormat=inherit  Unit=inherit  AffineConversion=off
  Conn1 : PMIOPort  Side=Left
  Conn2 : PMIOPort  Port=2  Side=Right
  output : Outport
  wires:
  PS-Simulink Converter1/1 -> output/1
  connections:
  Current Sensor1/RConn1 -- PS-Simulink Converter1/LConn1
  Current Sensor1/LConn1 -- Conn1/RConn1
  Current Sensor1/RConn2 -- Conn2/RConn1

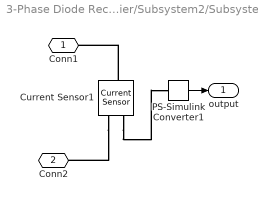
== system 3-Phase Diode Rectifier/Subsystem2/Subsystem2 ==
  Current Sensor1 : fl_lib/Electrical/Electrical Sensors/Current Sensor
  PS-Simulink Converter1 : nesl_utility/PS-Simulink Converter  PhysicalDomain=network_engine_domain  SubClassName=ps_output  LeftPortType=input  RightPortType=output  PseudoPeriodic=off  Frequencies=[]  VectorFormat=inherit  Unit=inherit  AffineConversion=off
  Conn1 : PMIOPort  Side=Left
  Conn2 : PMIOPort  Port=2  Side=Right
  output : Outport
  wires:
  PS-Simulink Converter1/1 -> output/1
  connections:
  Current Sensor1/RConn1 -- PS-Simulink Converter1/LConn1
  Current Sensor1/LConn1 -- Conn1/RConn1
  Current Sensor1/RConn2 -- Conn2/RConn1

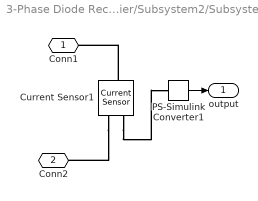
== system 3-Phase Diode Rectifier/Subsystem2/Subsystem3 ==
  Current Sensor1 : fl_lib/Electrical/Electrical Sensors/Current Sensor
  PS-Simulink Converter1 : nesl_utility/PS-Simulink Converter  PhysicalDomain=network_engine_domain  SubClassName=ps_output  LeftPortType=input  RightPortType=output  PseudoPeriodic=off  Frequencies=[]  VectorFormat=inherit  Unit=inherit  AffineConversion=off
  Conn1 : PMIOPort  Side=Left
  Conn2 : PMIOPort  Port=2  Side=Right
  output : Outport
  wires:
  PS-Simulink Converter1/1 -> output/1
  connections:
  Current Sensor1/RConn1 -- PS-Simulink Converter1/LConn1
  Current Sensor1/LConn1 -- Conn1/RConn1
  Current Sensor1/RConn2 -- Conn2/RConn1

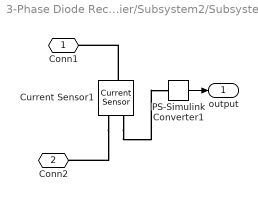
== system 3-Phase Diode Rectifier/Subsystem2/Subsystem4 ==
  Current Sensor1 : fl_lib/Electrical/Electrical Sensors/Current Sensor
  PS-Simulink Converter1 : nesl_utility/PS-Simulink Converter  PhysicalDomain=network_engine_domain  SubClassName=ps_output  LeftPortType=input  RightPortType=output  PseudoPeriodic=off  Frequencies=[]  VectorFormat=inherit  Unit=inherit  AffineConversion=off
  Conn1 : PMIOPort  Side=Left
  Conn2 : PMIOPort  Port=2  Side=Right
  output : Outport
  wires:
  PS-Simulink Converter1/1 -> output/1
  connections:
  Current Sensor1/RConn1 -- PS-Simulink Converter1/LConn1
  Current Sensor1/LConn1 -- Conn1/RConn1
  Current Sensor1/RConn2 -- Conn2/RConn1
